simulink model "mySimulationScheme"  (R2021a)
settings: Solver=VariableStepAuto  StartTime=0.0  StopTime=20  RelTol=1e-3
model workspace (MAT data in the model file):
  firstWarning = 1
  originalScenarioChecksum = 'C777D8D004E8227793BA6FB88E4AFE4A'
values from neighbouring files (symbols this model uses):
  A = [0 1 0;0 0 1;0 0 (-1/tau)]    [main.m]
  C = [0 1 0]    [main.m]
  h = 1    [main.m]
  lambda = 50    [main.m]
  Ts = 0.1    [main.m]
undefined symbols (not defined in the file or in its folder): driving, matlabshared
libraries: drivingscenarioandsensors x4, pid_lib x2
(part 3 of 3)

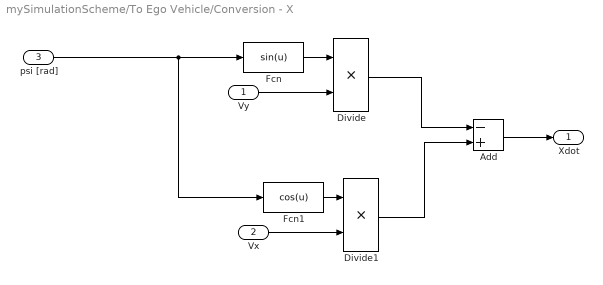
== system mySimulationScheme/To Ego Vehicle/Conversion - X ==
  Vy : Inport
  Vx : Inport  Port=2
  psi [rad] : Inport  Port=3
  Add : Sum  Inputs=-+
  Divide : Product  Inputs=**
  Divide1 : Product  Inputs=**
  Fcn : Fcn  Expr=sin(u)
  Fcn1 : Fcn  Expr=cos(u)
  Xdot : Outport
  wires:
  psi [rad]/1 -> Fcn/1, Fcn1/1
  Add/1 -> Xdot/1
  Divide1/1 -> Add/2
  Vx/1 -> Divide1/2
  Fcn1/1 -> Divide1/1
  Divide/1 -> Add/1
  Vy/1 -> Divide/2
  Fcn/1 -> Divide/1

== matlab function mySimulationScheme/Relevation Software/MATLAB Function1 ==
  data: radarSensor_1 input; x output; radarSensor_2 input; sensorCamera input; vx output; detections input; activation output
function [x,vx,activation] = getFromSensors(radarSensor_1,radarSensor_2,sensorCamera,detections)
% This Function Get The Relative Position & Velocity of Preceding Objects
measRadars      = zeros(6,1);
% Check The Presence Of Objects
if(detections(1) >= 1)
    % First Radar Detects Objects
    object           = radarSensor_1.Detections(1);
    % range rate measurements is enabled , so the state has 6 components
    measurements     = object.Measurement;
    measRadars(1)    = measurements(1);
    measRadars(2)    = measurements(4);
end
% From The Second Radar
if(detections(2) >= 1)
    % First Radar Detects Objects
    object           = radarSensor_2.Detections(1);
    % range rate measurements is enabled , so the state has 6 components
    measurements     = object.Measurement;
    measRadars(3)    = measurements(1);
    measRadars(4)    = measurements(4);
end
% From The Camera Sensor
if(detections(3) >= 1)
    % First Radar Detects Objects
    object           = sensorCamera.Detections(1);
    % range rate measurements is enabled , so the state has 6 components
    measurements     = object.Measurement;
    measRadars(5)    = measurements(1);
    measRadars(6)    = measurements(4);
end
% Take The Mean Value
x = (1/3)*(measRadars(1)+measRadars(3)+measRadars(5));
vx= (1/3)*(measRadars(2)+measRadars(4)+measRadars(6));
% Evaulate Activation
activation = detections;
end

== matlab function mySimulationScheme/Relevation Software/MATLAB Function ==
  data: radarSensor_1 input; detection output; radarSensor_2 input; sensorCamera input
function detection  = radarMeasurements(radarSensor_1,radarSensor_2,sensorCamera)
% This Function is able to detect objects from radar measurements
detection          = zeros(3,1);
% Check The Presence Of Objects from both radar sensors
% From First Radar
if(radarSensor_1.IsValidTime)
    detection(1)   = radarSensor_1.NumDetections;
end
% From Second Radar
if (radarSensor_2.IsValidTime)
    detection(2)   = radarSensor_2.NumDetections;
end
% From Camera Sensor
if (sensorCamera.IsValidTime)
    detection(3)   = sensorCamera.NumDetections;
end
end

== matlab function mySimulationScheme/To Ego Vehicle/MATLAB Function ==
  data: pos input; ego output Bus: BusActors1Actors; vel input
function ego = packEgo(pos,vel)
ego          = struct('ActorID',1,...
                      'Position',[pos -5.5047 0],...
                      'Velocity',[vel 0 0],...
                      'Roll',0,...
                      'Pitch',0,...
                      'Yaw',0,...
                      'AngularVelocity',[0 0 0]);
end

== matlab function mySimulationScheme/myACC/MATLAB Function ==
  data: activation input; enableCC output; enableDistC output; required input; relativePos input
function [enableCC,enableDistC] = getActivation(activation,required,relativePos)
% Of Course CC & ACC have to be in mutual esclusion
enableCC    = 0;
enableDistC = 0;
% The Activation of ACC is done by a relevation on an object
numDet      = sum(activation);
if(numDet >= 1)
      enableDistC = 1;
else
      enableCC    = 1;
end
end
